simulink model "general_bristle_model_1d"  (R2021b)
settings: Solver=FixedStepAuto  StartTime=0.0  StopTime=t_end  FixedStep=t_step  MaxStep=0.01  RelTol=1e-3  AbsTol=1e-3
undefined symbols (not defined in the file): d_1, d_2
libraries: fl_lib x7, nesl_utility x2
settings Model: Creator=Q657093  LastModifiedBy=q657093
settings SolverCC: AutoScaleAbsTol=off  ZeroCrossAlgorithm=Adaptive  AlgebraicLoopSolver=TrustRegion
settings DataIOCC: SaveFinalState=on  SaveState=on  InspectSignalLogs=on
settings DebuggingCC: IgnoredZcDiagnostic=none  SymbolicDimsDataTypeCodeGenerationDiagnostic=none
settings SFSimCC: CustomCodeUndefinedFunction=UseInterfaceOnly
settings SimscapeCC: ExplicitSolverDiagnosticOptions=none  SimscapeLogType=all  SimscapeLogSimulationStatistics=on  SimscapeLogToSDI=on  SimscapeLogDataHistory=10000

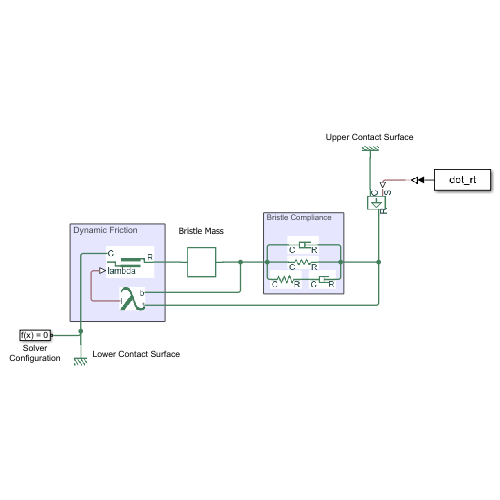
[thumbnail: Simulink's stored preview of the top-level diagram]
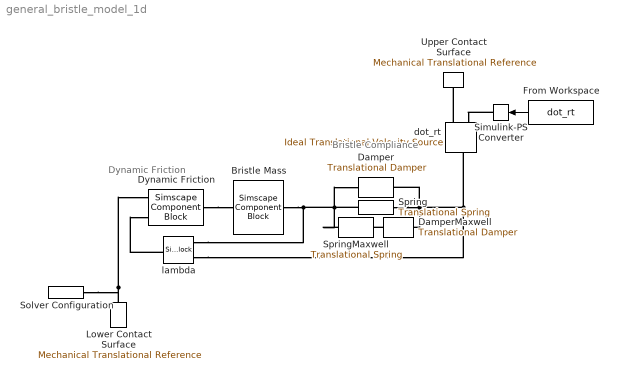
== system general_bristle_model_1d ==
  note: Bristle Compliance
  note: Dynamic Friction
  Bristle Mass : SimscapeComponentBlock  SourceFile=mass  ComponentPath=mass  ComponentVariants="[\"mass\"]"  ComponentVariantNames="[\"mass\"]"  ClassName=mass  SchemaVersion=1  mass=m_b kg  num_ports=foundation.enum.numPorts2.two  v_specify=on  v_priority=None  v=0 m/s  v_nominal_specify=off  v_nominal_unit=m/s  v_nominal_value=1  f_specify=off  f_priority=None  f=0 N  f_nominal_specify=off  f_nominal_unit=N  f_nominal_value=1
      settings: CopyFcn=simscape.engine.sli.internal.componentblockcallback(gcbh,'COPY')  PreCopyFcn=simscape.engine.sli.internal.componentblockcallback(gcbh,'PRECOPY')  PreDeleteFcn=simscape.engine.sli.internal.componentblockcallback(gcbh,'PREDELETE')  InternalSimscapePortConfiguration="{\"Bottom\":[],\"Left\":[{\"id\":\"M\",\"label\":\"\",\"type\":\"foundation.mechanical.translational.translational\"}],\"Right\":[{\"id\":\"N\",\"label\":\"\",\"type\":\"foundation.mechanical.translational.translational\"}],\"Top\":[]}"
      mask Type: Mass
  Damper : fl_lib/Mechanical/Translational Elements/Translational Damper  D=d_1 N/(m/s)  v_specify=off  v_priority=None  v=0 m/s  v_nominal_specify=off  v_nominal_unit=m/s  v_nominal_value=1  f_specify=off  f_priority=None  f=0 N  f_nominal_specify=off  f_nominal_unit=N  f_nominal_value=1
      settings: LogSimulationData=on
  DamperMaxwell : fl_lib/Mechanical/Translational Elements/Translational Damper  D=d_2 N/(m/s)  v_specify=off  v_priority=None  v=0 m/s  v_nominal_specify=off  v_nominal_unit=m/s  v_nominal_value=1  f_specify=off  f_priority=None  f=0 N  f_nominal_specify=off  f_nominal_unit=N  f_nominal_value=1
      settings: LogSimulationData=on
  Dynamic Friction : SimscapeComponentBlock  SourceFile=dynamic_friction  ComponentPath=dynamic_friction  ComponentVariants="[\"dynamic_friction\"]"  ComponentVariantNames="[\"dynamic_friction\"]"  ClassName=dynamic_friction  SchemaVersion=1  F_g=F_g N  F_h=F_h N  v_minslip=v_minslip m/s  lambda_flag=lambda_flag  v_specify=off  v_priority=None  v=0 m/s  v_nominal_specify=off  v_nominal_unit=m/s  v_nominal_value=1  f_specify=off  f_priority=None  f=0 N  f_nominal_specify=off  f_nominal_unit=N  f_nominal_value=1  stick_specify=off  stick_priority=None  stick=0
      settings: CopyFcn=simscape.engine.sli.internal.componentblockcallback(gcbh,'COPY')  PreCopyFcn=simscape.engine.sli.internal.componentblockcallback(gcbh,'PRECOPY')  PreDeleteFcn=simscape.engine.sli.internal.componentblockcallback(gcbh,'PREDELETE')  InternalSimscapePortConfiguration="{\"Bottom\":[],\"Left\":[{\"id\":\"R\",\"label\":\"R\",\"type\":\"foundation.mechanical.translational.translational\"}],\"Right\":[{\"id\":\"C\",\"label\":\"C\",\"type\":\"foundation.mechanical.translational.translational\"},{\"id\":\"lambda\",\"label\":\"lambda\",\"type\":\"input\"}],\"Top\":[]}"
      mask Type: Translational Friction
  From Workspace : FromWorkspace  VariableName=dot_rt  OutputAfterFinalValue=Holding final value
  Lower Contact Surface : fl_lib/Mechanical/Translational Elements/Mechanical Translational Reference
  Simulink-PS Converter : nesl_utility/Simulink-PS Converter  PhysicalDomain=network_engine_domain  SubClassName=ps_input  LeftPortType=input  RightPortType=output  PseudoPeriodic=off  Frequencies=[]  NoiseDistribution=none  NoiseParameters=[]  Unit=1  AffineConversion=off  FilteringAndDerivatives=provide  SimscapeFilterOrder=1  InputFilterTimeConstant=0.001  UdotUserProvided=0
      settings: SourceProductBaseCode=PW,SS
  Solver Configuration : nesl_utility/Solver Configuration  PhysicalDomain=network_engine_domain  SubClassName=solver  LeftPortType=input  RightPortType=generic  Tones=[]  Harmonics=[]  SimulateNoise=off  Profile=off  UseLocalSampling=off  EnableSwitchedLinearOptims=on  FrequencyDomain=off  UseCCode=off  RelTol=0.001  AbsTol=1e-06  MinStep=1e-09  ToWorkspace=off  RevertToSquareIcSolve=off  NumHomotopyIterations=100  PhasorMode=off  PhasorModeNumHarmonics=1  DoDC=off  ResidualTolerance=1e-09  UseLocalSolver=on  LocalSolverChoice=NE_BACKWARD_EULER_ADVANCER  LocalSolverSampleTime=0.001  DoFixedCost=on  MaxNonlinIter=3  MaxModeIter=2  ComputeImpulses=off  ImpulseIterations=2  LinearAlgebra=auto  EquationFormulation=NE_TIME_EF  DelaysMemoryBudget=1024  AutomaticFiltering=on  FilteringTimeConstant=0.001  PartitionStorageMethod=AS_NEEDED  PartitionMemoryBudget=1024  PartitionMethod=ROBUST
      settings: SourceProductBaseCode=PW,SS
  Spring : fl_lib/Mechanical/Translational Elements/Translational Spring  spr_rate=k_1 N/m  v_specify=off  v_priority=None  v=0 m/s  v_nominal_specify=off  v_nominal_unit=m/s  v_nominal_value=1  f_specify=off  f_priority=None  f=0 N  f_nominal_specify=off  f_nominal_unit=N  f_nominal_value=1  x_specify=off  x_priority=High  x=-0.1 m  x_nominal_specify=off  x_nominal_unit=m  x_nominal_value=1
  SpringMaxwell : fl_lib/Mechanical/Translational Elements/Translational Spring  spr_rate=k_2 N/m  v_specify=off  v_priority=None  v=0 m/s  v_nominal_specify=off  v_nominal_unit=m/s  v_nominal_value=1  f_specify=off  f_priority=None  f=0 N  f_nominal_specify=off  f_nominal_unit=N  f_nominal_value=1  x_specify=off  x_priority=High  x=-0.1 m  x_nominal_specify=off  x_nominal_unit=m  x_nominal_value=1
  Upper Contact Surface : fl_lib/Mechanical/Translational Elements/Mechanical Translational Reference
  dot_rt : fl_lib/Mechanical/Mechanical Sources/Ideal Translational Velocity Source
  lambda : SimscapeComponentBlock  SourceFile=lambda  ComponentPath=lambda  ComponentVariants="[\"lambda\"]"  ComponentVariantNames="[\"lambda\"]"  ClassName=lambda  SchemaVersion=1  F_g=F_g N  lambda_flag=lambda_flag
      settings: CopyFcn=simscape.engine.sli.internal.componentblockcallback(gcbh,'COPY')  PreCopyFcn=simscape.engine.sli.internal.componentblockcallback(gcbh,'PRECOPY')  PreDeleteFcn=simscape.engine.sli.internal.componentblockcallback(gcbh,'PREDELETE')  InternalSimscapePortConfiguration="{\"Bottom\":[],\"Left\":[{\"id\":\"top\",\"label\":\"t\",\"type\":\"foundation.mechanical.translational.translational\"},{\"id\":\"bottom\",\"label\":\"b\",\"type\":\"foundation.mechanical.translational.translational\"}],\"Right\":[{\"id\":\"l\",\"label\":\"l\",\"type\":\"output\"}],\"Top\":[]}"
      mask Type: lambda
  wires:
  From Workspace/1 -> Simulink-PS Converter/1
  connections:
  Bristle Mass/LConn1 -- SpringMaxwell/RConn1 -- Spring/RConn1 -- Damper/RConn1 -- lambda/LConn2
  dot_rt/RConn2 -- Upper Contact Surface/LConn1
  Simulink-PS Converter/RConn1 -- dot_rt/RConn1
  Dynamic Friction/LConn1 -- Bristle Mass/RConn1
  lambda/RConn1 -- Dynamic Friction/RConn2
  Lower Contact Surface/LConn1 -- Dynamic Friction/RConn1 -- Solver Configuration/RConn1
  lambda/LConn1 -- dot_rt/LConn1 -- Damper/LConn1 -- Spring/LConn1 -- DamperMaxwell/LConn1
  DamperMaxwell/RConn1 -- SpringMaxwell/LConn1
